simulink model "Alternator_Design"  (R2023b)
settings: Solver=ode23t  StartTime=0.0  StopTime=20  RelTol=1e-3
libraries: spsRMSLib x8, spsDCMachineLib x1, spsDCVoltageSourceLib x1, spsSynchronousMachineSIFundamentalLib x1, spsThreePhaseParallelRLCLoadLib x1, spsThreePhaseVIMeasurementLib x1, spsVoltageMeasurementLib x1, spspowerguiLib x1
settings Model: Creator=HP  LastModifiedBy=HP

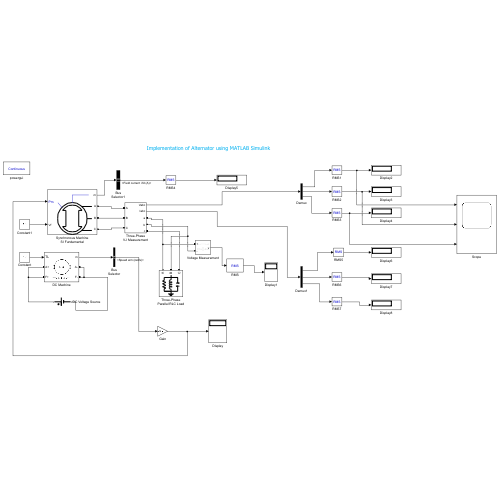
[thumbnail: Simulink's stored preview of the top-level diagram]
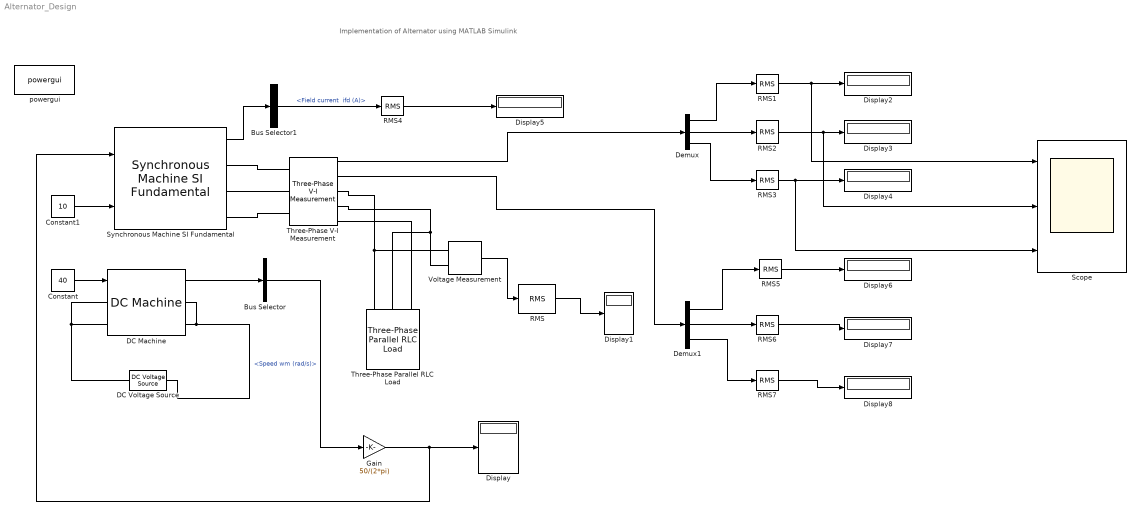
== system Alternator_Design ==
  note: Implementation of Alternator using MATLAB Simulink
  Bus Selector : BusSelector  OutputSignals=Speed wm (rad/s)
  Bus Selector1 : BusSelector  OutputSignals="dq0 components.Field current  ifd (A)"
  Constant : Constant  Value=40
  Constant1 : Constant  Value=10
  DC Machine : spsDCMachineLib/DC Machine  PresetModel=01: 5HP 240V 1750RPM Field:300V  MechanicalLoad=Torque TL  FieldType=Wound  ShowDetailedParameters=on  MeasurementBus=off  RLa=[2.581 0.028]  RLf=[281.2 156]  Laf=0.9483  MachineConstant=Torque constant (N.m/A)  Ke=1.8  Kt=1.8  J=0.02215  Bm=0.002953  Tf=0.5161  w0=1  Ifinit=0.85348506401138  TsPowergui=0  TsBlock=-1
  DC Voltage Source : spsDCVoltageSourceLib/DC Voltage Source  Amplitude=240  Measurements=None
  Demux : Demux  Outputs=3
  Demux1 : Demux  Outputs=3
  Display{,1..8} (9 alike) : Display
  Gain : Gain  Gain=50/(2*pi)
  RMS{,4..7} (5 alike) : spsRMSLib/RMS  TrueRMS=on  Freq=50  RMSInit=0  Ts=0.001
  RMS1 : spsRMSLib/RMS  TrueRMS=on  Freq=50  RMSInit=0  Ts=0.02
  RMS2 : spsRMSLib/RMS  TrueRMS=on  Freq=50  RMSInit=0  Ts=0.02
  RMS3 : spsRMSLib/RMS  TrueRMS=on  Freq=50  RMSInit=0  Ts=0.02
  Scope : Scope  NumInputPorts=3
  Synchronous Machine SI Fundamental : spsSynchronousMachineSIFundamentalLib/Synchronous Machine SI Fundamental  PresetModel=01: 50Hz 400V 8.1kVA 1500RPM  MechanicalLoad=Mechanical power Pm  ShowDetailedParameters=on  RotorType=Salient-pole  Units=SI fundamental parameters  MeasurementBus=off  NominalParameters=[8100 400 50]  Stator=[1.62 0.004527 0.1086 0.05175]  Field=[1.208 0.01132]  Dampers2=[ 0.0664, 1.387e-3, 0.0292, 6.896e-4, 7.907e-3, 2.477e-3]  Dampers1=[3.142 0.007334 4.772 0.01015]  Mechanical=[0.0923 0.009 2]  PolePairs=2  InitialConditions="[ 0  0  0  0  0  0  0  0  70.3192 ]"  SetSaturation=off  Saturation=[695.64,774.7,917.5,1001.6,1082.2,1175.9,1293.6,1430.2,1583.7;9660,10623,12243,13063,13757,14437,15180,15890,16567]  DisplayVfd=off  LoadFlowParameters=[1,0,0,0,0]  TsPowergui=0  TsBlock=-1  IterativeModel=Trapezoidal non iterative  IterativeDiscreteModel=Trapezoidal non iterative  BusType=PV  Pref=0  Qref=0  Qmin=-inf  Qmax=inf  PLF=0  QLF=0
      settings: LibrarySourceBlock=|
      | sps_lib/Electrical Machines/Synchronous Machine
      | SI Fundamental
  Three-Phase Parallel RLC Load : spsThreePhaseParallelRLCLoadLib/Three-Phase Parallel RLC Load  LConnTagsString=A|B|C  Configuration=Y (grounded)  NominalVoltage=6351  Vabc=[1e3 1e3 1e3]  Vabcp=[1e3 1e3 1e3]  NominalFrequency=50  UnbalancedPower=off  ActivePower=10e3  InductivePower=100  CapacitivePower=100  Pabc=[10e3 9e3 11e3]  QLabc=[100 90 110]  QCabc=[100 90 110]  Pabcp=[10e3 9e3 11e3]  QLabcp=[100 90 110]  QCabcp=[100 90 110]  Measurements=Branch voltages  LoadType=constant Z
  Three-Phase V-I Measurement : spsThreePhaseVIMeasurementLib/Three-Phase V-I Measurement  VoltageMeasurement=phase-to-ground  SetLabelV=off  LabelV=Vabc  Vpu=off  VpuLL=off  CurrentMeasurement=yes  SetLabelI=off  LabelI=Iabc  Ipu=off  Pbase=100e6  Vbase=500e3  OutputType=Complex  PhasorSimulation=off  PSBequivalent=0
  Voltage Measurement : spsVoltageMeasurementLib/Voltage Measurement  PhasorSimulation=off  OutputType=Complex  PSBequivalent=0
  powergui : spspowerguiLib/powergui  Priority=1  SimulationMode=Continuous  SampleTime=50e-6  frequency=60  Iterations=50  frequencyindice=50  Pbase=100e6  ErrMax=1e-4  UnitsV=kV  UnitsW=MW  buscounter=0  FunctionMessages=off  echomessages=off  EnableUseOfTLC=off  CurrentSourceSwitches=off  DisableSnubberDevices=off  DisableRonSwitches=off  DisableVfSwitches=off  DisplayEquations=off  AutomaticDiscreteSolvers=off  SolverType=Tustin/Backward Euler (TBE)  Interpol=off  ExternalGateDelay=off  methode=off  Ts=100  x0status=blocks  SPID=on  SwTol=0  HookPort=off  NonlinearTolerance=1e-4  nMaxIteration=100  ContinueOnMaxIteration=off  RestoreLinks=warning  ResistiveCurrentMeasurement=off  Frange=[0:2:500]  Ylog=off  Xlog=on  ShowGrid=off  save=off  variable=ZData  structure=0  ZoomFFT=off  StartTime=0.0  cycles=1  DisplayStyle=1  fundamental=60  FreqAxis=off  MaxFrequency=1000  frequencyindicesteady=1  RmsSteady=1  display=off
  wires:
  Constant/1 -> DC Machine/1
  DC Machine/1 -> Bus Selector/1
  Bus Selector/1 -> Gain/1  "<Speed wm (rad/s)>"
  Gain/1 -> Synchronous Machine SI Fundamental/1, Display/1
  Constant1/1 -> Synchronous Machine SI Fundamental/2
  Voltage Measurement/1 -> RMS/1
  RMS/1 -> Display1/1
  Three-Phase V-I Measurement/1 -> Demux/1
  Demux/1 -> RMS1/1
  Demux/2 -> RMS2/1
  Demux/3 -> RMS3/1
  RMS1/1 -> Scope/1, Display2/1
  RMS2/1 -> Scope/2, Display3/1
  RMS3/1 -> Scope/3, Display4/1
  Synchronous Machine SI Fundamental/1 -> Bus Selector1/1
  Bus Selector1/1 -> RMS4/1  "<Field current  ifd (A)>"
  RMS4/1 -> Display5/1
  Three-Phase V-I Measurement/2 -> Demux1/1
  Demux1/1 -> RMS5/1
  Demux1/2 -> RMS6/1
  Demux1/3 -> RMS7/1
  RMS5/1 -> Display6/1
  RMS6/1 -> Display7/1
  RMS7/1 -> Display8/1
  connections:
  DC Machine/LConn2 -- DC Voltage Source/RConn1 -- DC Machine/LConn1
  DC Machine/RConn2 -- DC Machine/RConn1 -- DC Voltage Source/LConn1
  Three-Phase V-I Measurement/LConn1 -- Synchronous Machine SI Fundamental/RConn1
  Three-Phase V-I Measurement/LConn2 -- Synchronous Machine SI Fundamental/RConn2
  Three-Phase V-I Measurement/LConn3 -- Synchronous Machine SI Fundamental/RConn3
  Three-Phase Parallel RLC Load/LConn1 -- Three-Phase V-I Measurement/RConn1 -- Voltage Measurement/LConn1
  Three-Phase Parallel RLC Load/LConn2 -- Three-Phase V-I Measurement/RConn2 -- Voltage Measurement/LConn2
  Three-Phase Parallel RLC Load/LConn3 -- Three-Phase V-I Measurement/RConn3
